simulink model "MPM_v1"  (R2018b)
settings: Solver=VariableStepAuto  StartTime=0.0  StopTime=10.0  RelTol=1e-3
undefined symbols (not defined in the file): Cw, Cwc, Jt, Jw, k1, k2, k3, k4, Mt, R3, R4, Rg, Rw
settings Model: Creator=HYJ  LastModifiedBy=HYJ

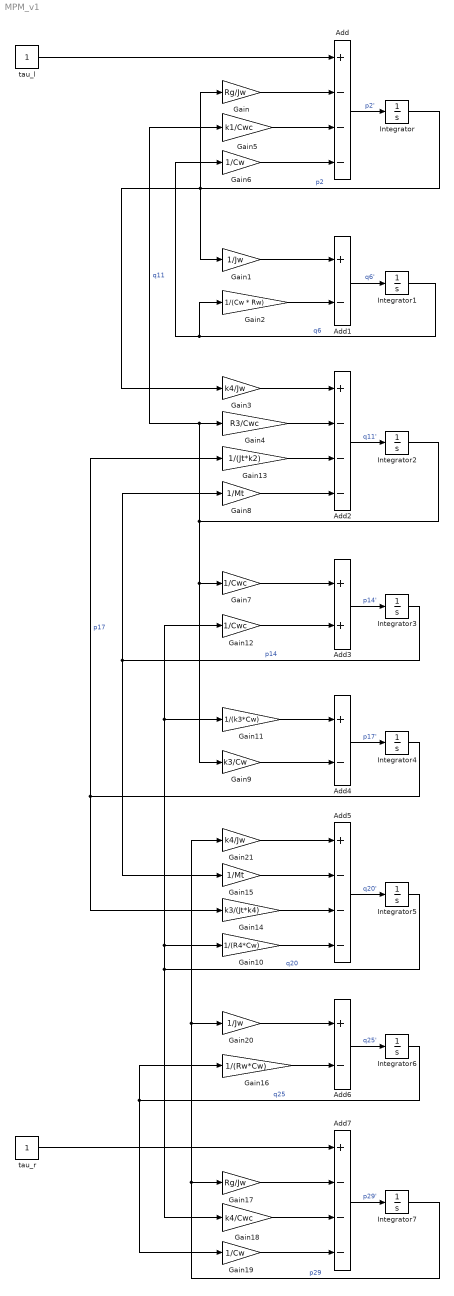
== system MPM_v1 ==
  Add{,2,5,7} (4 alike) : Sum  Inputs=+---
  Add1 : Sum  Inputs=+-
  Add3 : Sum
  Add4 : Sum  Inputs=+-
  Add6 : Sum  Inputs=+-
  Gain : Gain  Gain=Rg/Jw
  Gain1 : Gain  Gain=1/Jw
  Gain10 : Gain  Gain=1/(R4*Cw)
  Gain11 : Gain  Gain=1/(k3*Cw)
  Gain12 : Gain  Gain=1/Cwc
  Gain13 : Gain  Gain=1/(Jt*k2)
  Gain14 : Gain  Gain=k3/(Jt*k4)
  Gain15 : Gain  Gain=1/Mt
  Gain16 : Gain  Gain=1/(Rw*Cw)
  Gain17 : Gain  Gain=Rg/Jw
  Gain18 : Gain  Gain=k4/Cwc
  Gain19 : Gain  Gain=1/Cw
  Gain2 : Gain  Gain=1/(Cw * Rw)
  Gain20 : Gain  Gain=1/Jw
  Gain21 : Gain  Gain=k4/Jw
  Gain3 : Gain  Gain=k4/Jw
  Gain4 : Gain  Gain=R3/Cwc
  Gain5 : Gain  Gain=k1/Cwc
  Gain6 : Gain  Gain=1/Cw
  Gain7 : Gain  Gain=1/Cwc
  Gain8 : Gain  Gain=1/Mt
  Gain9 : Gain  Gain=k3/Cw
  Integrator{,1..7} (8 alike) : Integrator
  tau_l : Constant
  tau_r : Constant
  wires:
  tau_l/1 -> Add/1
  Add/1 -> Integrator/1  "p2'"
  Integrator/1 -> Gain3/1, Gain1/1, Gain/1  "p2"
  Gain/1 -> Add/2
  Gain1/1 -> Add1/1
  Add1/1 -> Integrator1/1  "q6'"
  Gain2/1 -> Add1/2
  Integrator1/1 -> Gain6/1, Gain2/1  "q6"
  Add2/1 -> Integrator2/1  "q11'"
  Gain3/1 -> Add2/1
  Gain4/1 -> Add2/2
  Integrator2/1 -> Gain9/1, Gain7/1, Gain5/1, Gain4/1  "q11"
  Gain5/1 -> Add/3
  Gain6/1 -> Add/4
  Add3/1 -> Integrator3/1  "p14'"
  Gain7/1 -> Add3/1
  Integrator3/1 -> Gain8/1, Gain15/1  "p14"
  Gain8/1 -> Add2/4
  Add4/1 -> Integrator4/1  "p17'"
  Gain9/1 -> Add4/2
  Add5/1 -> Integrator5/1  "q20'"
  Gain10/1 -> Add5/4
  Integrator5/1 -> Gain10/1, Gain12/1, Gain11/1, Gain18/1  "q20"
  Gain11/1 -> Add4/1
  Gain12/1 -> Add3/2
  Integrator4/1 -> Gain13/1, Gain14/1  "p17"
  Gain13/1 -> Add2/3
  Gain14/1 -> Add5/3
  Gain15/1 -> Add5/2
  Add6/1 -> Integrator6/1  "q25'"
  Gain16/1 -> Add6/2
  Integrator6/1 -> Gain19/1, Gain16/1  "q25"
  Gain18/1 -> Add7/3
  Integrator7/1 -> Gain21/1, Gain20/1, Gain17/1  "p29"
  Gain19/1 -> Add7/4
  tau_r/1 -> Add7/1
  Gain17/1 -> Add7/2
  Add7/1 -> Integrator7/1  "p29'"
  Gain20/1 -> Add6/1
  Gain21/1 -> Add5/1
